simulink library "imu_block_visual"  (R2025b)
settings: Solver=VariableStepAuto  StartTime=0.0  StopTime=10.0  RelTol=1e-3
undefined symbols (not defined in the file or in its folder): ADXL, IMU, Sim
settings Model: Creator=Ashwin  LastModifiedBy=Ashwin

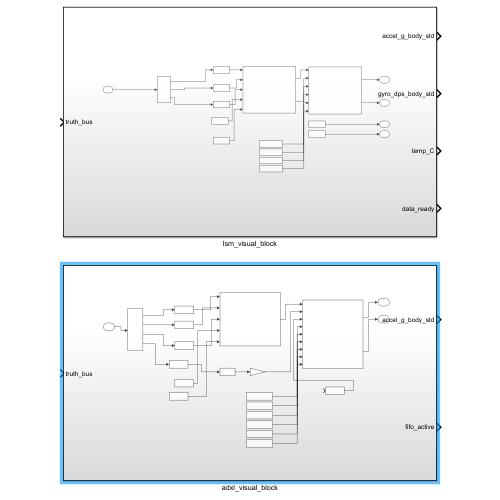
[thumbnail: Simulink's stored preview of the top-level diagram]
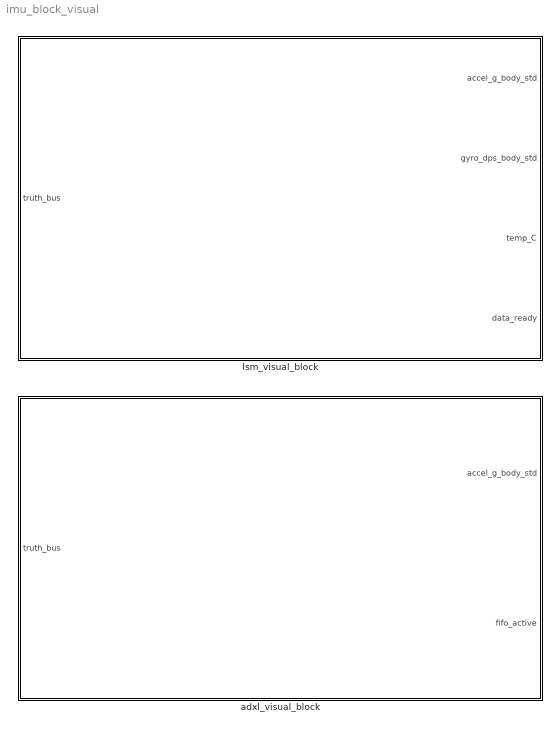
== system imu_block_visual ==
  adxl_visual_block : Subsystem
  lsm_visual_block : Subsystem

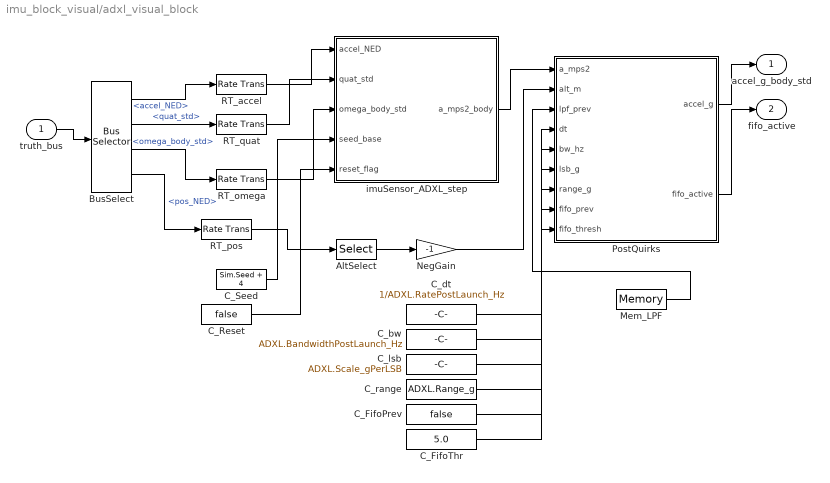
== system imu_block_visual/adxl_visual_block ==
  truth_bus : Inport  OutDataTypeStr=Bus: SensorInputBus
  AltSelect : Selector  InputPortWidth=3  IndexOptions=Index vector (dialog)  Indices=3  OutputSizes=1
  BusSelect : BusSelector  OutputSignals=accel_NED,quat_std,omega_body_std,pos_NED
  C_FifoPrev : Constant  Value=false  OutDataTypeStr=boolean  SampleTime=1/ADXL.RatePostLaunch_Hz
  C_FifoThr : Constant  Value=5.0  SampleTime=1/ADXL.RatePostLaunch_Hz
  C_Reset : Constant  Value=false  OutDataTypeStr=boolean  SampleTime=1/ADXL.RatePostLaunch_Hz
  C_Seed : Constant  Value=Sim.Seed + 4  SampleTime=1/ADXL.RatePostLaunch_Hz
  C_bw : Constant  Value=ADXL.BandwidthPostLaunch_Hz  SampleTime=1/ADXL.RatePostLaunch_Hz
  C_dt : Constant  Value=1/ADXL.RatePostLaunch_Hz  SampleTime=1/ADXL.RatePostLaunch_Hz
  C_lsb : Constant  Value=ADXL.Scale_gPerLSB  SampleTime=1/ADXL.RatePostLaunch_Hz
  C_range : Constant  Value=ADXL.Range_g  SampleTime=1/ADXL.RatePostLaunch_Hz
  Mem_LPF : Memory  InitialCondition=[0; 0; 0]
  NegGain : Gain  Gain=-1
  PostQuirks : MATLAB Function  TreatAsAtomicUnit=on
  RT_accel : RateTransition  OutPortSampleTime=1/ADXL.RatePostLaunch_Hz
  RT_omega : RateTransition  OutPortSampleTime=1/ADXL.RatePostLaunch_Hz
  RT_pos : RateTransition  OutPortSampleTime=1/ADXL.RatePostLaunch_Hz
  RT_quat : RateTransition  OutPortSampleTime=1/ADXL.RatePostLaunch_Hz
  imuSensor_ADXL_step : MATLAB Function  TreatAsAtomicUnit=on
  accel_g_body_std : Outport
  fifo_active : Outport  Port=2
  wires:
  truth_bus/1 -> BusSelect/1
  BusSelect/1 -> RT_accel/1  "<accel_NED>"
  BusSelect/2 -> RT_quat/1  "<quat_std>"
  BusSelect/3 -> RT_omega/1  "<omega_body_std>"
  BusSelect/4 -> RT_pos/1  "<pos_NED>"
  RT_pos/1 -> AltSelect/1
  AltSelect/1 -> NegGain/1
  RT_accel/1 -> imuSensor_ADXL_step/1(accel_NED)
  RT_quat/1 -> imuSensor_ADXL_step/2(quat_std)
  RT_omega/1 -> imuSensor_ADXL_step/3(omega_body_std)
  C_Seed/1 -> imuSensor_ADXL_step/4(seed_base)
  C_Reset/1 -> imuSensor_ADXL_step/5(reset_flag)
  imuSensor_ADXL_step/1(a_mps2_body) -> PostQuirks/1(a_mps2)
  NegGain/1 -> PostQuirks/2(alt_m)
  Mem_LPF/1 -> PostQuirks/3(lpf_prev)
  C_dt/1 -> PostQuirks/4(dt)
  C_bw/1 -> PostQuirks/5(bw_hz)
  C_lsb/1 -> PostQuirks/6(lsb_g)
  C_range/1 -> PostQuirks/7(range_g)
  C_FifoPrev/1 -> PostQuirks/8(fifo_prev)
  C_FifoThr/1 -> PostQuirks/9(fifo_thresh)
  PostQuirks/1(accel_g) -> accel_g_body_std/1
  PostQuirks/2(fifo_active) -> fifo_active/1

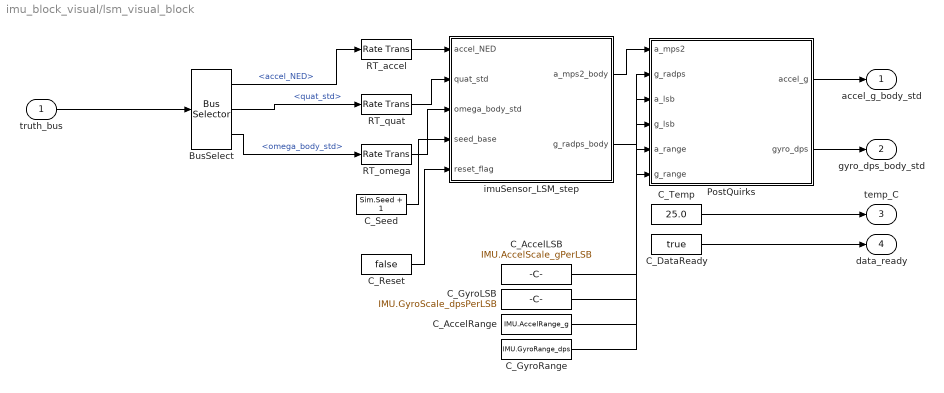
== system imu_block_visual/lsm_visual_block ==
  truth_bus : Inport  OutDataTypeStr=Bus: SensorInputBus
  BusSelect : BusSelector  OutputSignals=accel_NED,quat_std,omega_body_std
  C_AccelLSB : Constant  Value=IMU.AccelScale_gPerLSB  SampleTime=1/IMU.Rate_Hz
  C_AccelRange : Constant  Value=IMU.AccelRange_g  SampleTime=1/IMU.Rate_Hz
  C_DataReady : Constant  Value=true  OutDataTypeStr=boolean  SampleTime=1/IMU.Rate_Hz
  C_GyroLSB : Constant  Value=IMU.GyroScale_dpsPerLSB  SampleTime=1/IMU.Rate_Hz
  C_GyroRange : Constant  Value=IMU.GyroRange_dps  SampleTime=1/IMU.Rate_Hz
  C_Reset : Constant  Value=false  OutDataTypeStr=boolean  SampleTime=1/IMU.Rate_Hz
  C_Seed : Constant  Value=Sim.Seed + 1  SampleTime=1/IMU.Rate_Hz
  C_Temp : Constant  Value=25.0  SampleTime=1/IMU.Rate_Hz
  PostQuirks : MATLAB Function  TreatAsAtomicUnit=on
  RT_accel : RateTransition  OutPortSampleTime=1/IMU.Rate_Hz
  RT_omega : RateTransition  OutPortSampleTime=1/IMU.Rate_Hz
  RT_quat : RateTransition  OutPortSampleTime=1/IMU.Rate_Hz
  imuSensor_LSM_step : MATLAB Function  TreatAsAtomicUnit=on
  accel_g_body_std : Outport
  gyro_dps_body_std : Outport  Port=2
  temp_C : Outport  Port=3
  data_ready : Outport  Port=4
  wires:
  truth_bus/1 -> BusSelect/1
  BusSelect/1 -> RT_accel/1  "<accel_NED>"
  BusSelect/2 -> RT_quat/1  "<quat_std>"
  BusSelect/3 -> RT_omega/1  "<omega_body_std>"
  RT_accel/1 -> imuSensor_LSM_step/1(accel_NED)
  RT_quat/1 -> imuSensor_LSM_step/2(quat_std)
  RT_omega/1 -> imuSensor_LSM_step/3(omega_body_std)
  C_Seed/1 -> imuSensor_LSM_step/4(seed_base)
  C_Reset/1 -> imuSensor_LSM_step/5(reset_flag)
  imuSensor_LSM_step/1(a_mps2_body) -> PostQuirks/1(a_mps2)
  imuSensor_LSM_step/2(g_radps_body) -> PostQuirks/2(g_radps)
  C_AccelLSB/1 -> PostQuirks/3(a_lsb)
  C_GyroLSB/1 -> PostQuirks/4(g_lsb)
  C_AccelRange/1 -> PostQuirks/5(a_range)
  C_GyroRange/1 -> PostQuirks/6(g_range)
  PostQuirks/1(accel_g) -> accel_g_body_std/1
  PostQuirks/2(gyro_dps) -> gyro_dps_body_std/1
  C_Temp/1 -> temp_C/1
  C_DataReady/1 -> data_ready/1

== matlab function imu_block_visual/lsm_visual_block/PostQuirks ==
  data: a_mps2 input; accel_g output; g_radps input; a_lsb input; g_lsb input; a_range input; g_range input; gyro_dps output
function [accel_g, gyro_dps] = fcn(a_mps2, g_radps, a_lsb, g_lsb, a_range, g_range)
%#codegen
[accel_g, gyro_dps] = casper_imu_lsm_quirks(a_mps2(:), g_radps(:), a_lsb, g_lsb, a_range, g_range);
end

== matlab function imu_block_visual/lsm_visual_block/imuSensor_LSM_step ==
  data: accel_NED input; a_mps2_body output; quat_std input; omega_body_std input; seed_base input; reset_flag input; g_radps_body output
function [a_mps2_body, g_radps_body] = fcn(accel_NED, quat_std, omega_body_std, seed_base, reset_flag)
coder.extrinsic('casper_imu_lsm_step');
a_mps2_body = zeros(1,3); g_radps_body = zeros(1,3);
[a_mps2_body, g_radps_body, ~] = casper_imu_lsm_step(accel_NED(:).', omega_body_std(:).', quat_std(:).', double(seed_base), logical(reset_flag));
end

== matlab function imu_block_visual/adxl_visual_block/imuSensor_ADXL_step ==
  data: accel_NED input; a_mps2_body output; quat_std input; omega_body_std input; seed_base input; reset_flag input
function a_mps2_body = fcn(accel_NED, quat_std, omega_body_std, seed_base, reset_flag)
coder.extrinsic('casper_imu_adxl_step');
a_mps2_body = zeros(1,3);
a_mps2_body = casper_imu_adxl_step(accel_NED(:).', omega_body_std(:).', quat_std(:).', double(seed_base), logical(reset_flag));
end

== matlab function imu_block_visual/adxl_visual_block/PostQuirks ==
  data: a_mps2 input; accel_g output; alt_m input; lpf_prev input; dt input; bw_hz input; lsb_g input; range_g input; fifo_prev input; fifo_thresh input; fifo_active output
function [accel_g, fifo_active] = fcn(a_mps2, alt_m, lpf_prev, dt, bw_hz, lsb_g, range_g, fifo_prev, fifo_thresh)
%#codegen
[accel_g, ~, fifo_active] = casper_imu_adxl_quirks(a_mps2(:), lpf_prev(:), alt_m, dt, bw_hz, lsb_g, range_g, logical(fifo_prev), fifo_thresh);
end
